simulink model "Drone_Simulink_Model_v2"  (R2020b)
settings: Solver=VariableStepAuto  StartTime=0.0  StopTime=10  RelTol=1e-3
PreLoadFcn:
  | InitialConditions
values from neighbouring files (symbols this model uses):
  AmpsHour = 1.8    [InitialConditions.m]
  b_m = 2.415*10^-6    (= 2.415e-06)    [InitialConditions.m]
  Discharge = 80    [InitialConditions.m]
  Jr_v = 6.5*10^-7    (= 6.5e-07)    [InitialConditions.m]
  Kemf = 0.00255    [InitialConditions.m]
  Kt = 0.00255    [InitialConditions.m]
  L_ind = 1.17*10^-4    (= 0.000117)    [InitialConditions.m]
  R = 0.117    [InitialConditions.m]
  u_1 = 2*pi*rpm_mot1/60    (= 104.71975512)    [InitialConditions.m]
  u_2 = 2*pi*rpm_mot2/60    (= 104.71975512)    [InitialConditions.m]
  u_3 = 2*pi*rpm_mot3/60    (= 104.71975512)    [InitialConditions.m]
  u_4 = 2*pi*rpm_mot4/60    (= 104.71975512)    [InitialConditions.m]
  v0 = [0 ... (first row only)    [InitialConditions.m]
  x0 = [0 ... (first row only)    [InitialConditions.m]
undefined symbols (not defined in the file or in its folder): DRONE_MODEL, Transformation
libraries: simulink x5, pid_lib x4, aerolibutil x2, vrlib x1
settings Model: Creator=kelep  LastModifiedBy=kelep

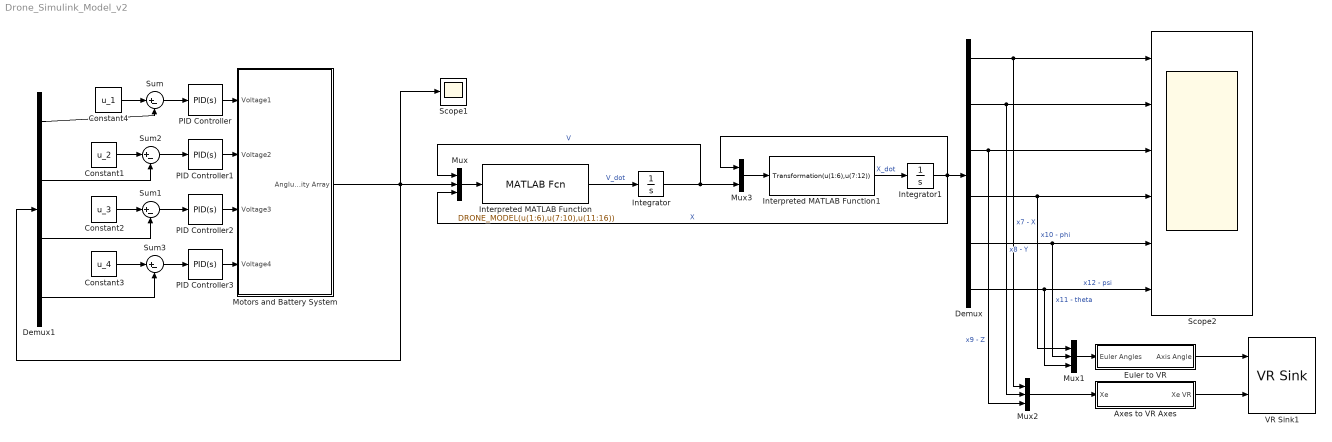
== system Drone_Simulink_Model_v2 ==
  Axes to VR Axes : Subsystem
  Constant1 : Constant  Value=u_2
  Constant2 : Constant  Value=u_3
  Constant3 : Constant  Value=u_4
  Constant4 : Constant  Value=u_1
  Demux : Demux  Outputs=6
  Demux1 : Demux
  Euler to VR : Subsystem
  Integrator : Integrator  InitialCondition=v0
  Integrator1 : Integrator  InitialCondition=x0
  Interpreted MATLAB Function : MATLABFcn  MATLABFcn=DRONE_MODEL(u(1:6),u(7:10),u(11:16))
  Interpreted MATLAB Function1 : MATLABFcn  MATLABFcn=Transformation(u(1:6),u(7:12))
  Motors and Battery System : Subsystem
  Mux : Mux  Inputs=3
  Mux1 : Mux  Inputs=3
  Mux2 : Mux  Inputs=3
  Mux3 : Mux  Inputs=2
  PID Controller{,1..3} (4 alike) : pid_lib/PID Controller  Controller=PID  Form=Parallel  TimeDomain=Continuous-time  UseExternalTs=off  SampleTime=-1  IntegratorMethod=Forward Euler  FilterMethod=Forward Euler  ControllerParametersSource=internal  P=1  I=0  D=0  UseFilter=on  N=100  TunerSelectOption=Transfer Function Based (PID Tuner App)  InitialConditionSource=internal  InitialConditionForIntegrator=0  InitialConditionForFilter=0  DifferentiatorICPrevScaledInput=0  ExternalReset=none  TrackingMode=off  Kt=1  LimitOutput=off  SatLimitsSource=internal  UpperSaturationLimit=inf  LowerSaturationLimit=-inf  LinearizeAsGain=on  AntiWindupMode=none  Kb=1  POutMin=[]  POutMax=[]  IOutMin=[]  IOutMax=[]  DOutMin=[]  DOutMax=[]  NOutMin=[]  NOutMax=[]  SumOutMin=[]  SumOutMax=[]  SaturationOutMin=[]  SaturationOutMax=[]  PParamMin=[]  PParamMax=[]  IParamMin=[]  IParamMax=[]  DParamMin=[]  DParamMax=[]  NParamMin=[]  NParamMax=[]  KbParamMin=[]  KbParamMax=[]  KtParamMin=[]  KtParamMax=[]  KbOutMin=[]  KbOutMax=[]  KtOutMin=[]  KtOutMax=[]  IntegratorOutMin=[]  IntegratorOutMax=[]  FilterOutMin=[]  FilterOutMax=[]  SumI1OutMin=[]  SumI1OutMax=[]  SumI2OutMin=[]  SumI2OutMax=[]  SumI3OutMin=[]  SumI3OutMax=[]  SumI4OutMin=[]  SumI4OutMax=[]  SumDOutMin=[]  SumDOutMax=[]  DifferentiatorOutMin=[]  DifferentiatorOutMax=[]  FilterDiffOutCoefMin=[]  FilterDiffOutCoefMax=[]  ReciprocalOutMin=[]  ReciprocalOutMax=[]  SumDenOutMin=[]  SumDenOutMax=[]  SumNumOutMin=[]  SumNumOutMax=[]  DivideOutMin=[]  DivideOutMax=[]  UdiffTsProdOutMin=[]  UdiffTsProdOutMax=[]  NTsProdOutMin=[]  NTsProdOutMax=[]  UintegralTsProdOutMin=[]  UintegralTsProdOutMax=[]  UngainTsProdOutMin=[]  UngainTsProdOutMax=[]  IntegratorContinuousStateAttributes=''  IntegratorStateMustResolveToSignalObject=off  IntegratorRTWStateStorageClass=Auto  FilterContinuousStateAttributes=''  FilterStateMustResolveToSignalObject=off  FilterRTWStateStorageClass=Auto  ParallelPVariant=InternalParameters  IdealPVariant=Disabled  IVariant=InternalParameters  DVariant=InternalParameters  IntegratorVariant=Continuous  SatVariant=Disabled  AWVariant=Passthrough  PCopyVariant=Disabled  TRVariant=Disabled  FdbkBlocksVariant=Forward  IdealPFdbkVariant=Disabled  SatFdbkVariant=Disabled  DerivativeFilterVariant=ContFilter  NVariant=InternalParameters  NCopyVariant=Disabled  FilterICVariant=InternalICsFilter  IntegratorICVariant=InternalICs  ExternalResetVariant=Disabled  TRSumVariant=Passthrough  SumFdbkVariant=Disabled  SumVariant=Sum_PID  TsampFilterVariant=InternalTs  TsampNgainVariant=Passthrough  TsampIntegralVariant=Passthrough  ExternalSaturationOutDataTypeStr=Inherit: Same as second input
  Scope1 : Scope
  Scope2 : Scope  NumInputPorts=6
  Sum{,1..3} (4 alike) : Sum  Inputs=|+-
  VR Sink1 : vrlib/VR Sink  InstantiateOnLoad=on  SampleTime=0.1  ViewEnable=on  RemoteChange=off  RemoteView=off  FieldsWritten=HL20.rotation.4.1.1.double#HL20.translation.3.1.1.double  WorldFileName=aeroblk_HL20.wrl  WorldDescription=aeroblk_HL20  AutoView=on  VideoDimensions=[]  AllowVariableSize=off
  wires:
  Interpreted MATLAB Function/1 -> Integrator/1  "V_dot"
  Mux/1 -> Interpreted MATLAB Function/1
  Integrator/1 -> Mux3/2, Mux/1  "V"
  Motors and Battery System/1(Anglular Velocity Array) -> Mux/2, Scope1/1, Demux1/1
  PID Controller/1 -> Motors and Battery System/1(Voltage1)
  PID Controller2/1 -> Motors and Battery System/3(Voltage3)
  PID Controller1/1 -> Motors and Battery System/2(Voltage2)
  PID Controller3/1 -> Motors and Battery System/4("Voltage4 ")
  Constant1/1 -> Sum2/1
  Constant2/1 -> Sum1/1
  Constant3/1 -> Sum3/1
  Sum/1 -> PID Controller/1
  Sum3/1 -> PID Controller3/1
  Sum2/1 -> PID Controller1/1
  Sum1/1 -> PID Controller2/1
  Demux1/1 -> Sum/2
  Demux1/2 -> Sum2/2
  Demux1/3 -> Sum1/2
  Demux1/4 -> Sum3/2
  Constant4/1 -> Sum/1
  Demux/1 -> Scope2/1, Mux2/1  "x7 - X"
  Demux/2 -> Mux2/2, Scope2/2  "x8 - Y"
  Demux/3 -> Mux2/3, Scope2/3  "x9 - Z"
  Demux/4 -> Mux1/1, Scope2/4  "x10 - phi"
  Demux/5 -> Mux1/2, Scope2/5  "x11 - theta"
  Demux/6 -> Mux1/3, Scope2/6  "x12 - psi"
  Euler to VR/1(Axis Angle) -> VR Sink1/1
  Mux2/1 -> Axes to VR Axes/1(Xe)
  Axes to VR Axes/1(Xe VR) -> VR Sink1/2
  Mux1/1 -> Euler to VR/1(Euler Angles)
  Mux3/1 -> Interpreted MATLAB Function1/1
  Interpreted MATLAB Function1/1 -> Integrator1/1  "X_dot"
  Integrator1/1 -> Mux/3, Mux3/1, Demux/1  "X"

== system Drone_Simulink_Model_v2/Axes to VR Axes ==
  Xe : Inport
  Concatenate : Concatenate  NumInputs=3
  Demux : Demux  Outputs=3
      settings: DisplayOption=none
  rad-->deg : Gain  Gain=-1  SaturateOnIntegerOverflow=on  OutDataTypeStr=Inherit: Same as input  ParamDataTypeStr=Inherit: Same as input
  rad-->deg1 : Gain  Gain=-1  SaturateOnIntegerOverflow=on  OutDataTypeStr=Inherit: Same as input  ParamDataTypeStr=Inherit: Same as input
  Xe VR : Outport  VectorParamsAs1DForOutWhenUnconnected=off
  wires:
  Xe/1 -> Demux/1
  Demux/1 -> Concatenate/1
  Demux/2 -> rad-->deg/1
  Demux/3 -> rad-->deg1/1
  Concatenate/1 -> Xe VR/1
  rad-->deg1/1 -> Concatenate/2
  rad-->deg/1 -> Concatenate/3

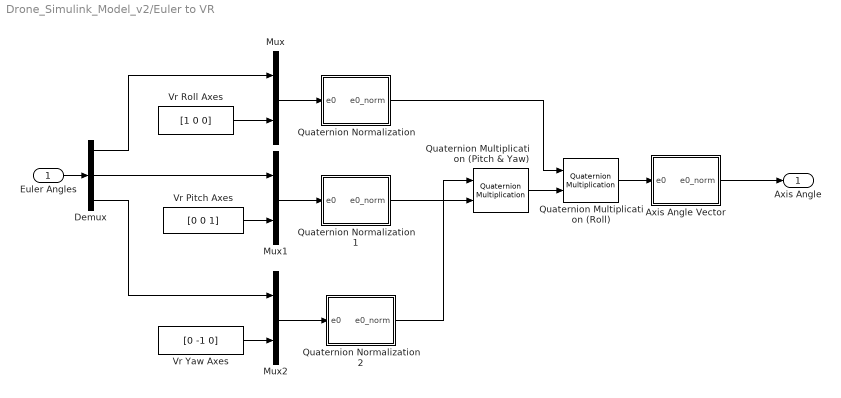
== system Drone_Simulink_Model_v2/Euler to VR ==
  Euler Angles : Inport
  Axis Angle Vector : Subsystem
  Demux : Demux  Outputs=3
      settings: DisplayOption=none
  Mux : Mux  Inputs=2
  Mux1 : Mux  Inputs=2
  Mux2 : Mux  Inputs=2
  Quaternion Multiplication (Pitch & Yaw) : aerolibutil/Quaternion Multiplication
  Quaternion Multiplication (Roll) : aerolibutil/Quaternion Multiplication
  Quaternion Normalization : Subsystem
  Quaternion Normalization1 : Subsystem
  Quaternion Normalization2 : Subsystem
  Vr Pitch Axes : Constant  Value=[0 0 1]
  Vr Roll Axes : Constant  Value=[1 0 0]
  Vr Yaw Axes : Constant  Value=[0 -1 0]
  Axis Angle : Outport  VectorParamsAs1DForOutWhenUnconnected=off
  wires:
  Quaternion Multiplication (Roll)/1 -> Axis Angle Vector/1(e0)
  Quaternion Multiplication (Pitch & Yaw)/1 -> Quaternion Multiplication (Roll)/2
  Axis Angle Vector/1(e0_norm) -> Axis Angle/1
  Quaternion Normalization/1(e0_norm) -> Quaternion Multiplication (Roll)/1
  Quaternion Normalization2/1(e0_norm) -> Quaternion Multiplication (Pitch & Yaw)/1
  Quaternion Normalization1/1(e0_norm) -> Quaternion Multiplication (Pitch & Yaw)/2
  Mux2/1 -> Quaternion Normalization2/1(e0)
  Mux1/1 -> Quaternion Normalization1/1(e0)
  Mux/1 -> Quaternion Normalization/1(e0)
  Demux/3 -> Mux2/1
  Vr Yaw Axes/1 -> Mux2/2
  Demux/2 -> Mux1/1
  Vr Pitch Axes/1 -> Mux1/2
  Demux/1 -> Mux/1
  Vr Roll Axes/1 -> Mux/2
  Euler Angles/1 -> Demux/1

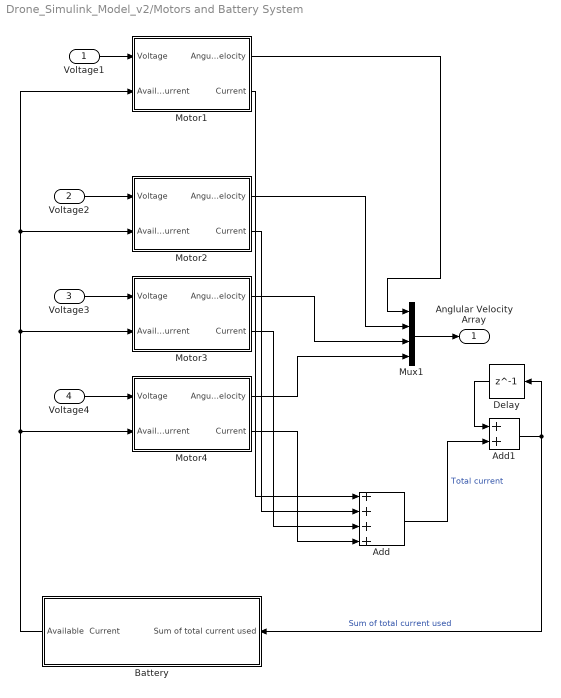
== system Drone_Simulink_Model_v2/Motors and Battery System ==
  Voltage1 : Inport
  Voltage2 : Inport  Port=2
  Voltage3 : Inport  Port=3
  "Voltage4 " : Inport  Port=4
  Add : Sum  Inputs=++++
  Add1 : Sum
  Battery : Subsystem
  Delay : Delay  DelayLength=1  SampleTime=0.01
  Motor1 : Subsystem
  Motor2 : Subsystem
  Motor3 : Subsystem
  Motor4 : Subsystem
  Mux1 : Mux
  Anglular Velocity Array : Outport
  wires:
  Voltage3/1 -> Motor3/1(Voltage)
  Motor2/2("Current ") -> Add/2
  Motor4/1("Angular Velocity ") -> Mux1/4
  Motor2/1("Angular Velocity ") -> Mux1/2
  Voltage2/1 -> Motor2/1(Voltage)
  Voltage1/1 -> Motor1/1("Voltage ")
  Add/1 -> Add1/2  "Total current"
  Motor1/2("Current ") -> Add/1
  Motor3/2("Current ") -> Add/3
  Motor4/2("Current ") -> Add/4
  Motor3/1("Angular Velocity ") -> Mux1/3
  Motor1/1("Angular Velocity ") -> Mux1/1
  "Voltage4 "/1 -> Motor4/1(Voltage)
  Mux1/1 -> Anglular Velocity Array/1
  Add1/1 -> Delay/1, Battery/1(Sum of total current used)  "Sum of total current used"
  Battery/1(Available  Current) -> Motor4/2(Available Current), Motor1/2("Availble Current "), Motor2/2("Available Current "), Motor3/2(Available Current)
  Delay/1 -> Add1/1

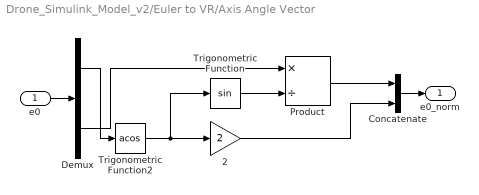
== system Drone_Simulink_Model_v2/Euler to VR/Axis Angle Vector ==
  e0 : Inport
  2 : Gain  Gain=2  SaturateOnIntegerOverflow=on  OutDataTypeStr=Inherit: Same as input  ParamDataTypeStr=Inherit: Same as input
  Concatenate : Concatenate
  Demux : Demux  Outputs=[1 3 ]
      settings: DisplayOption=none
  Product : Product  Inputs=*/  InputSameDT=on  SaturateOnIntegerOverflow=on  OutDataTypeStr=Inherit: Same as first input
  Trigonometric Function : Trigonometry
  Trigonometric Function2 : Trigonometry  Operator=acos
  e0_norm : Outport  VectorParamsAs1DForOutWhenUnconnected=off
  wires:
  Demux/1 -> Trigonometric Function2/1
  Demux/2 -> Product/1
  Concatenate/1 -> e0_norm/1
  Product/1 -> Concatenate/1
  2/1 -> Concatenate/2
  Trigonometric Function/1 -> Product/2
  Trigonometric Function2/1 -> Trigonometric Function/1, 2/1
  e0/1 -> Demux/1

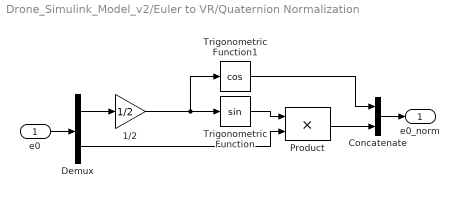
== system Drone_Simulink_Model_v2/Euler to VR/Quaternion Normalization ==
  e0 : Inport
  1/2 : Gain  Gain=1/2  SaturateOnIntegerOverflow=on  OutDataTypeStr=Inherit: Same as input  ParamDataTypeStr=Inherit: Same as input
  Concatenate : Concatenate
  Demux : Demux  Outputs=[1 3]
      settings: DisplayOption=none
  Product : Product  InputSameDT=on  SaturateOnIntegerOverflow=on  OutDataTypeStr=Inherit: Same as first input
  Trigonometric Function : Trigonometry
  Trigonometric Function1 : Trigonometry  Operator=cos
  e0_norm : Outport  VectorParamsAs1DForOutWhenUnconnected=off
  wires:
  Trigonometric Function1/1 -> Concatenate/1
  Demux/2 -> Product/2
  Demux/1 -> 1/2/1
  Concatenate/1 -> e0_norm/1
  Product/1 -> Concatenate/2
  Trigonometric Function/1 -> Product/1
  1/2/1 -> Trigonometric Function1/1, Trigonometric Function/1
  e0/1 -> Demux/1

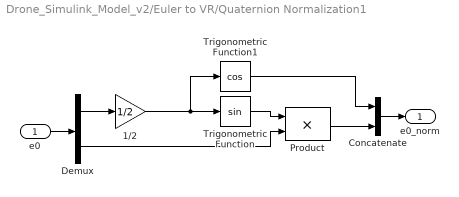
== system Drone_Simulink_Model_v2/Euler to VR/Quaternion Normalization1 ==
  e0 : Inport
  1/2 : Gain  Gain=1/2  SaturateOnIntegerOverflow=on  OutDataTypeStr=Inherit: Same as input  ParamDataTypeStr=Inherit: Same as input
  Concatenate : Concatenate
  Demux : Demux  Outputs=[1 3]
      settings: DisplayOption=none
  Product : Product  InputSameDT=on  SaturateOnIntegerOverflow=on  OutDataTypeStr=Inherit: Same as first input
  Trigonometric Function : Trigonometry
  Trigonometric Function1 : Trigonometry  Operator=cos
  e0_norm : Outport  VectorParamsAs1DForOutWhenUnconnected=off
  wires:
  e0/1 -> Demux/1
  1/2/1 -> Trigonometric Function/1, Trigonometric Function1/1
  Trigonometric Function/1 -> Product/1
  Product/1 -> Concatenate/2
  Concatenate/1 -> e0_norm/1
  Demux/1 -> 1/2/1
  Demux/2 -> Product/2
  Trigonometric Function1/1 -> Concatenate/1

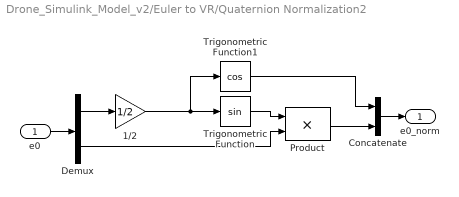
== system Drone_Simulink_Model_v2/Euler to VR/Quaternion Normalization2 ==
  e0 : Inport
  1/2 : Gain  Gain=1/2  SaturateOnIntegerOverflow=on  OutDataTypeStr=Inherit: Same as input  ParamDataTypeStr=Inherit: Same as input
  Concatenate : Concatenate
  Demux : Demux  Outputs=[1 3]
      settings: DisplayOption=none
  Product : Product  InputSameDT=on  SaturateOnIntegerOverflow=on  OutDataTypeStr=Inherit: Same as first input
  Trigonometric Function : Trigonometry
  Trigonometric Function1 : Trigonometry  Operator=cos
  e0_norm : Outport  VectorParamsAs1DForOutWhenUnconnected=off
  wires:
  Trigonometric Function1/1 -> Concatenate/1
  Demux/2 -> Product/2
  Demux/1 -> 1/2/1
  Concatenate/1 -> e0_norm/1
  Product/1 -> Concatenate/2
  Trigonometric Function/1 -> Product/1
  1/2/1 -> Trigonometric Function1/1, Trigonometric Function/1
  e0/1 -> Demux/1

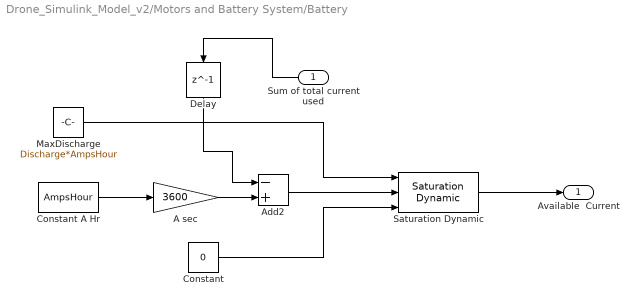
== system Drone_Simulink_Model_v2/Motors and Battery System/Battery ==
  Sum of total current used : Inport
  A sec : Gain  Gain=3600
  Add2 : Sum  Inputs=-+
  Constant : Constant  Value=0
  Constant A Hr : Constant  Value=AmpsHour
  Delay : Delay  DelayLength=1  SampleTime=0.01
  MaxDischarge : Constant  Value=Discharge*AmpsHour
  Saturation Dynamic : simulink/Discontinuities/Saturation Dynamic  OutMin=[]  OutMax=[]  OutDataTypeStr=Inherit: Same as second input  OutDataType=fixdt(1, 16)  OutScaling=2^-10  DoSatur=off
  Available  Current : Outport
  wires:
  Sum of total current used/1 -> Delay/1
  A sec/1 -> Add2/2
  Add2/1 -> Saturation Dynamic/2
  Saturation Dynamic/1 -> Available  Current/1
  Constant A Hr/1 -> A sec/1
  MaxDischarge/1 -> Saturation Dynamic/1
  Constant/1 -> Saturation Dynamic/3
  Delay/1 -> Add2/1

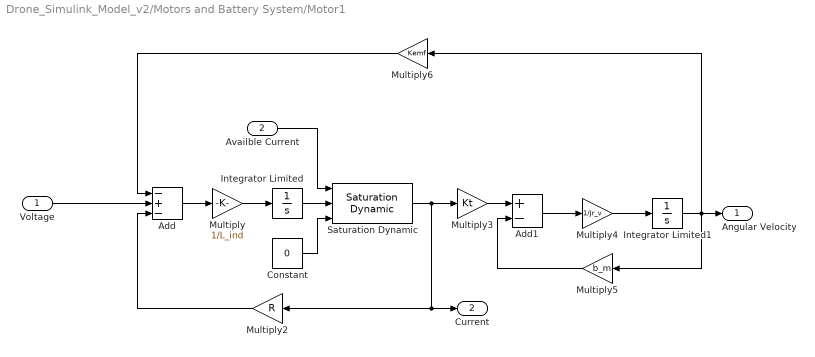
== system Drone_Simulink_Model_v2/Motors and Battery System/Motor1 ==
  "Voltage " : Inport
  "Availble Current " : Inport  Port=2
  Add : Sum  Inputs=-+-
  Add1 : Sum  Inputs=+-
  Constant : Constant  Value=0
  Integrator Limited : Integrator  LimitOutput=on  UpperSaturationLimit=20  LowerSaturationLimit=0
  Integrator Limited1 : Integrator  LimitOutput=on  UpperSaturationLimit=300  LowerSaturationLimit=0
  Multiply : Gain  Gain=1/L_ind
  Multiply2 : Gain  Gain=R
  Multiply3 : Gain  Gain=Kt
  Multiply4 : Gain  Gain=1/Jr_v
  Multiply5 : Gain  Gain=b_m
  Multiply6 : Gain  Gain=Kemf
  Saturation Dynamic : simulink/Discontinuities/Saturation Dynamic  OutMin=[]  OutMax=[]  OutDataTypeStr=Inherit: Same as second input  OutDataType=fixdt(1, 16)  OutScaling=2^-10  DoSatur=off
  "Angular Velocity " : Outport
  "Current " : Outport  Port=2
  wires:
  Multiply3/1 -> Add1/1
  Multiply/1 -> Integrator Limited/1
  Integrator Limited1/1 -> Multiply5/1, Multiply6/1, "Angular Velocity "/1
  Add/1 -> Multiply/1
  Multiply5/1 -> Add1/2
  Add1/1 -> Multiply4/1
  Multiply2/1 -> Add/3
  Multiply6/1 -> Add/1
  Multiply4/1 -> Integrator Limited1/1
  "Voltage "/1 -> Add/2
  Integrator Limited/1 -> Saturation Dynamic/2
  Saturation Dynamic/1 -> Multiply2/1, "Current "/1, Multiply3/1
  Constant/1 -> Saturation Dynamic/3
  "Availble Current "/1 -> Saturation Dynamic/1

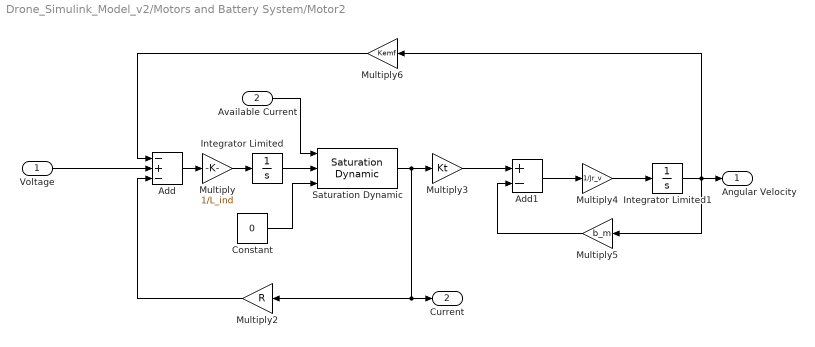
== system Drone_Simulink_Model_v2/Motors and Battery System/Motor2 ==
  Voltage : Inport
  "Available Current " : Inport  Port=2
  Add : Sum  Inputs=-+-
  Add1 : Sum  Inputs=+-
  Constant : Constant  Value=0
  Integrator Limited : Integrator  LimitOutput=on  UpperSaturationLimit=20  LowerSaturationLimit=0
  Integrator Limited1 : Integrator  LimitOutput=on  UpperSaturationLimit=300  LowerSaturationLimit=0
  Multiply : Gain  Gain=1/L_ind
  Multiply2 : Gain  Gain=R
  Multiply3 : Gain  Gain=Kt
  Multiply4 : Gain  Gain=1/Jr_v
  Multiply5 : Gain  Gain=b_m
  Multiply6 : Gain  Gain=Kemf
  Saturation Dynamic : simulink/Discontinuities/Saturation Dynamic  OutMin=[]  OutMax=[]  OutDataTypeStr=Inherit: Same as second input  OutDataType=fixdt(1, 16)  OutScaling=2^-10  DoSatur=off
  "Angular Velocity " : Outport
  "Current " : Outport  Port=2
  wires:
  Multiply3/1 -> Add1/1
  Multiply/1 -> Integrator Limited/1
  Integrator Limited1/1 -> Multiply5/1, Multiply6/1, "Angular Velocity "/1
  Add/1 -> Multiply/1
  Multiply5/1 -> Add1/2
  Add1/1 -> Multiply4/1
  Multiply2/1 -> Add/3
  Multiply6/1 -> Add/1
  Multiply4/1 -> Integrator Limited1/1
  Voltage/1 -> Add/2
  Integrator Limited/1 -> Saturation Dynamic/2
  Saturation Dynamic/1 -> "Current "/1, Multiply2/1, Multiply3/1
  Constant/1 -> Saturation Dynamic/3
  "Available Current "/1 -> Saturation Dynamic/1

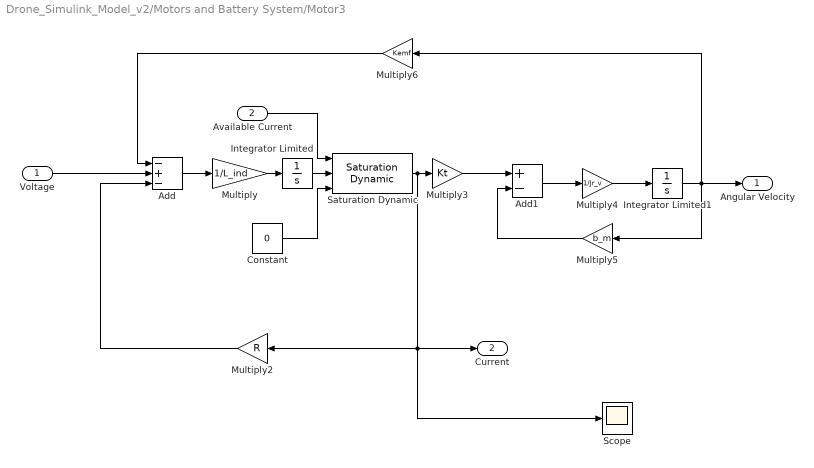
== system Drone_Simulink_Model_v2/Motors and Battery System/Motor3 ==
  Voltage : Inport
  Available Current : Inport  Port=2
  Add : Sum  Inputs=-+-
  Add1 : Sum  Inputs=+-
  Constant : Constant  Value=0
  Integrator Limited : Integrator  LimitOutput=on  UpperSaturationLimit=20  LowerSaturationLimit=0
  Integrator Limited1 : Integrator  LimitOutput=on  UpperSaturationLimit=300  LowerSaturationLimit=0
  Multiply : Gain  Gain=1/L_ind
  Multiply2 : Gain  Gain=R
  Multiply3 : Gain  Gain=Kt
  Multiply4 : Gain  Gain=1/Jr_v
  Multiply5 : Gain  Gain=b_m
  Multiply6 : Gain  Gain=Kemf
  Saturation Dynamic : simulink/Discontinuities/Saturation Dynamic  OutMin=[]  OutMax=[]  OutDataTypeStr=Inherit: Same as second input  OutDataType=fixdt(1, 16)  OutScaling=2^-10  DoSatur=off
  Scope : Scope
  "Angular Velocity " : Outport
  "Current " : Outport  Port=2
  wires:
  Multiply3/1 -> Add1/1
  Multiply/1 -> Integrator Limited/1
  Integrator Limited/1 -> Saturation Dynamic/2
  Integrator Limited1/1 -> Multiply5/1, Multiply6/1, "Angular Velocity "/1
  Add/1 -> Multiply/1
  Multiply5/1 -> Add1/2
  Add1/1 -> Multiply4/1
  Multiply2/1 -> Add/3
  Multiply6/1 -> Add/1
  Multiply4/1 -> Integrator Limited1/1
  Voltage/1 -> Add/2
  Saturation Dynamic/1 -> Scope/1, Multiply2/1, "Current "/1, Multiply3/1
  Constant/1 -> Saturation Dynamic/3
  Available Current/1 -> Saturation Dynamic/1

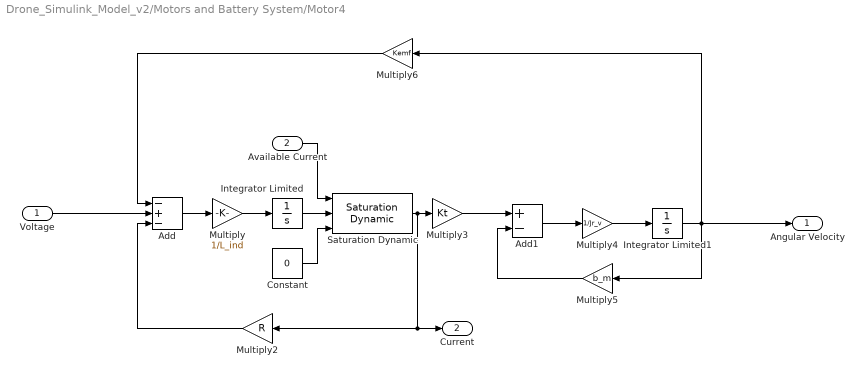
== system Drone_Simulink_Model_v2/Motors and Battery System/Motor4 ==
  Voltage : Inport
  Available Current : Inport  Port=2
  Add : Sum  Inputs=-+-
  Add1 : Sum  Inputs=+-
  Constant : Constant  Value=0
  Integrator Limited : Integrator  LimitOutput=on  UpperSaturationLimit=20  LowerSaturationLimit=0
  Integrator Limited1 : Integrator  LimitOutput=on  UpperSaturationLimit=300  LowerSaturationLimit=0
  Multiply : Gain  Gain=1/L_ind
  Multiply2 : Gain  Gain=R
  Multiply3 : Gain  Gain=Kt
  Multiply4 : Gain  Gain=1/Jr_v
  Multiply5 : Gain  Gain=b_m
  Multiply6 : Gain  Gain=Kemf
  Saturation Dynamic : simulink/Discontinuities/Saturation Dynamic  OutMin=[]  OutMax=[]  OutDataTypeStr=Inherit: Same as second input  OutDataType=fixdt(1, 16)  OutScaling=2^-10  DoSatur=off
  "Angular Velocity " : Outport
  "Current " : Outport  Port=2
  wires:
  Multiply3/1 -> Add1/1
  Multiply/1 -> Integrator Limited/1
  Integrator Limited1/1 -> Multiply5/1, Multiply6/1, "Angular Velocity "/1
  Add/1 -> Multiply/1
  Multiply5/1 -> Add1/2
  Add1/1 -> Multiply4/1
  Multiply2/1 -> Add/3
  Multiply6/1 -> Add/1
  Multiply4/1 -> Integrator Limited1/1
  Voltage/1 -> Add/2
  Saturation Dynamic/1 -> Multiply2/1, "Current "/1, Multiply3/1
  Integrator Limited/1 -> Saturation Dynamic/2
  Constant/1 -> Saturation Dynamic/3
  Available Current/1 -> Saturation Dynamic/1
